simulink model "hybridperes (2)"  (R2019a)
settings: Solver=VariableStepAuto  StartTime=0.0  StopTime=10.0  RelTol=1e-3
libraries: powerlib x28, re_lib x2, powerlib_meascontrol x2
settings Model: Creator=USER  LastModifiedBy=USER

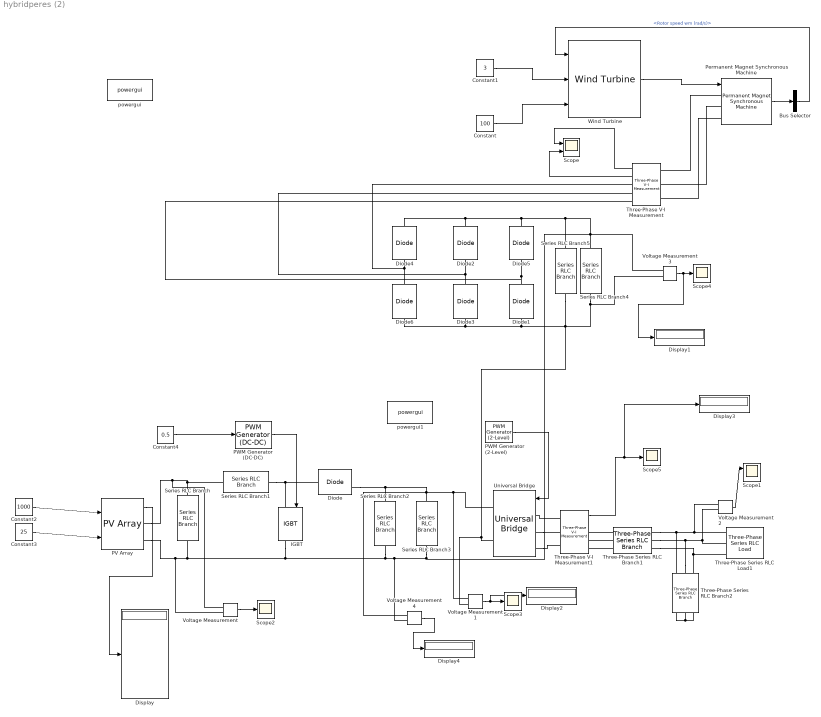
== system hybridperes (2) ==
  Bus Selector : BusSelector  OutputSignals=Rotor speed wm (rad/s)
  Constant : Constant  Value=100
  Constant1 : Constant  Value=3
  Constant2 : Constant  Value=1000
  Constant3 : Constant  Value=25
  Constant4 : Constant  Value=0.5
  Diode : powerlib/Power Electronics/Diode  Ron=0.001  Lon=0  Vf=0.8  IC=0  UseSnubber=0  Rs=500  Cs=250e-9  Measurements=on
      settings: SourceProductName=Simscape Electrical
  Diode{1..6} (6 alike) : powerlib/Power Electronics/Diode  Ron=0.001  Lon=0  Vf=0.8  IC=0  UseSnubber=0  Rs=500  Cs=250e-9  Measurements=off
      settings: SourceProductName=Simscape Electrical
  Display{,1..4} (5 alike) : Display
  IGBT : powerlib/Power Electronics/IGBT  Ron=0.001  Lon=0  Vf=1  Tf=1e-6  Tt=2e-6  IC=0  Rs=1e5  Cs=inf  Measurements=on
      settings: SourceProductName=Simscape Electrical
  PV Array : re_lib/Solar/PV Array  Npar=4  Nser=1  PlotType=array @ 1000 W/m2 & specified temperatures  S_vec="[ 1000  500  100 ]"  Temp_C_vec="[ 45 25  ]"  ModuleName=User-defined  PlotWhenSelected=off  Pm=213.15  Ncell=60  Voc=36.3  Isc=7.84  Vm=29  Im=7.35  beta_Voc_pc=-0.36099  alpha_Isc_pc=0.102  beta_Voc=-0.13104  alpha_Isc=0.0079968  IL=7.8654  I0=2.9273e-10  nI=0.98119  Rsh=313.0553  Rs=0.39381  BAL=on  Tc=1e-6  Tfilter=5e-5
      settings: SourceProductName=Simscape Electrical
  PWM Generator (2-Level) : powerlib_meascontrol/Pulse & Signal Generators/PWM Generator (2-Level)  ModulatorType=Three-phase bridge (6 pulses)  ModulatorMode=Unsynchronized  Fc=27*50*3  Pc=90  nF=27  MinMax="[ -1  1 ]"  SamplingTechnique=Natural  ModulatingSignals=on  m=0.8  Freq=50  Phase=0  Ts=0  ShowCarrierOutport=off
  PWM Generator (DC-DC) : powerlib_meascontrol/Pulse & Signal Generators/PWM Generator (DC-DC)  Fsw=5000  Ts=0
      settings: SourceProductName=Simscape Electrical
  Permanent Magnet Synchronous Machine : powerlib/Machines/Permanent Magnet Synchronous Machine  NbPhases=3  FluxDistribution=Sinusoidal  RotorType=Round  MechanicalLoad=Torque Tm  PresetModel=No  ShowDetailedParameters=on  MeasurementBus=off  Resistance=0.0485  Inductance=8.5e-3  dqInductances=[8.5e-3,8.5e-3]  La=0.000395  MachineConstant=Flux linkage established by magnets (V.s)  Flux=0.1194  VoltageCst=86.6271  TorqueCst=0.7164  Flat=120  Mechanical=[0.0027 0.0004924 4 0]  PolePairs=4  InitialConditions=[0,0, 0,0]  InitialConditions5ph=[0 0 0 0 0 0]  TsPowergui=0  TsBlock=-1  RefAngle=90 degrees behind phase A axis (modified Park)
  Scope : Scope  NumInputPorts=2
  Scope1 : Scope  NumInputPorts=2
  Scope{2..5} (4 alike) : Scope
  Series RLC Branch : powerlib/Elements/Series RLC Branch  LConnTagsString=__new0  RConnTagsString=__new0  BranchType=C  Resistance=1  Inductance=1e-3  SetiL0=off  InitialCurrent=0  Capacitance=0.5  Setx0=off  InitialVoltage=0  Measurements=None
      settings: SourceProductName=Simscape Electrical
  Series RLC Branch1 : powerlib/Elements/Series RLC Branch  LConnTagsString=__new0  RConnTagsString=__new0  BranchType=L  Resistance=1  Inductance=160e-6  SetiL0=off  InitialCurrent=0  Capacitance=1e-6  Setx0=off  InitialVoltage=0  Measurements=None
      settings: SourceProductName=Simscape Electrical
  Series RLC Branch2 : powerlib/Elements/Series RLC Branch  LConnTagsString=__new0  RConnTagsString=__new0  BranchType=C  Resistance=1  Inductance=1e-3  SetiL0=off  InitialCurrent=0  Capacitance=83e-3  Setx0=off  InitialVoltage=0  Measurements=None
      settings: SourceProductName=Simscape Electrical
  Series RLC Branch3 : powerlib/Elements/Series RLC Branch  LConnTagsString=__new0  RConnTagsString=__new0  BranchType=R  Resistance=2  Inductance=1e-3  SetiL0=off  InitialCurrent=0  Capacitance=1e-6  Setx0=off  InitialVoltage=0  Measurements=None
      settings: SourceProductName=Simscape Electrical
  Series RLC Branch4 : powerlib/Elements/Series RLC Branch  LConnTagsString=__new0  RConnTagsString=__new0  BranchType=R  Resistance=1  Inductance=1e-3  SetiL0=off  InitialCurrent=0  Capacitance=1e-6  Setx0=off  InitialVoltage=0  Measurements=None
      settings: SourceProductName=Simscape Electrical
  Series RLC Branch5 : powerlib/Elements/Series RLC Branch  LConnTagsString=__new0  RConnTagsString=__new0  BranchType=C  Resistance=1  Inductance=1e-3  SetiL0=off  InitialCurrent=0  Capacitance=10e-3  Setx0=off  InitialVoltage=0  Measurements=None
      settings: SourceProductName=Simscape Electrical
  Three-Phase Series RLC Branch1 : powerlib/Elements/Three-Phase Series RLC Branch  LConnTagsString=A|B|C  RConnTagsString=A|B|C  BranchType=L  Resistance=1  Inductance=0.001023  Capacitance=1e-6  Measurements=None
      settings: SourceProductName=Simscape Electrical
  Three-Phase Series RLC Branch2 : powerlib/Elements/Three-Phase Series RLC Branch  LConnTagsString=A|B|C  RConnTagsString=A|B|C  BranchType=C  Resistance=1  Inductance=1e-3  Capacitance=0.008456  Measurements=None
      settings: SourceProductName=Simscape Electrical
  Three-Phase Series RLC Load1 : powerlib/Elements/Three-Phase Series RLC Load  LConnTagsString=A|B|C  Configuration=Y (grounded)  NominalVoltage=1000  Vabc=[1e3 1e3 1e3]  Vabcp=[1e3 1e3 1e3]  NominalFrequency=50  UnbalancedPower=off  ActivePower=10e3  InductivePower=0  CapacitivePower=0  Pabc=[10e3 9e3 11e3]  QLabc=[100 90 110]  QCabc=[100 90 110]  Pabcp=[10e3 9e3 11e3]  QLabcp=[100 90 110]  QCabcp=[100 90 110]  Measurements=None  LoadType=constant Z
      settings: SourceProductName=Simscape Electrical
  Three-Phase V-I Measurement : powerlib/Measurements/Three-Phase V-I Measurement  VoltageMeasurement=phase-to-phase  SetLabelV=off  LabelV=Vabc  Vpu=off  VpuLL=off  CurrentMeasurement=yes  SetLabelI=off  LabelI=Iabc  Ipu=off  Pbase=100e6  Vbase=500e3  OutputType=Complex  PhasorSimulation=off  PSBequivalent=0
      settings: SourceProductName=Simscape Electrical
  Three-Phase V-I Measurement1 : powerlib/Measurements/Three-Phase V-I Measurement  VoltageMeasurement=phase-to-ground  SetLabelV=off  LabelV=Vabc  Vpu=off  VpuLL=off  CurrentMeasurement=yes  SetLabelI=off  LabelI=Iabc  Ipu=off  Pbase=100e6  Vbase=500e3  OutputType=Complex  PhasorSimulation=off  PSBequivalent=0
      settings: SourceProductName=Simscape Electrical
  Universal Bridge : powerlib/Power Electronics/Universal Bridge  Arms=3  SnubberResistance=1e5  SnubberCapacitance=inf  Device=IGBT / Diodes  Ron=1e-3  Lon=0  ForwardVoltages="[  0  0  ]"  ForwardVoltage=0  GTOparameters=[ 10e-6 , 20e-6 ]  IGBTparameters=[ 1e-6 , 2e-6 ]  Measurements=None  Measurements_2=None  converterType=Rectifier
      settings: SourceProductName=Simscape Electrical
  Voltage Measurement{,1..4} (5 alike) : powerlib/Measurements/Voltage Measurement  PhasorSimulation=off  OutputType=Complex  PSBequivalent=0
      settings: SourceProductName=Simscape Electrical
  Wind Turbine : re_lib/Wind Generation/Wind Turbine  Pnom=1.5e6  Pelec_base=1.5e6/0.9  wind_base=12  P_wind_base=0.73  speed_nom=1.2  pitch_angle=0  c1_c6="[0.51763          116          0.4            5           21     0.006795]"  cp_nom=0.48  lambda_nom=8.1
      settings: SourceProductName=Simscape Electrical  SourceProductBaseCode=PS
  powergui : powerlib/powergui  Priority=1  SimulationMode=Discrete  SampleTime=50e-6  frequency=60  Iterations=50  frequencyindice=0  Pbase=100e6  ErrMax=1e-4  UnitsV=kV  UnitsW=MW  buscounter=0  FunctionMessages=off  echomessages=off  EnableUseOfTLC=off  CurrentSourceSwitches=off  DisableSnubberDevices=off  DisableRonSwitches=off  DisableVfSwitches=off  DisplayEquations=off  AutomaticDiscreteSolvers=off  SolverType=Tustin/Backward Euler (TBE)  Interpol=off  ExternalGateDelay=off  methode=off  Ts=100  x0status=blocks  SPID=on  SwTol=0  HookPort=off  NonlinearTolerance=0  nMaxIteration=15  ContinueOnMaxIteration=off  RestoreLinks=warning  ResistiveCurrentMeasurement=off  Frange=[0:2:500]  Ylog=off  Xlog=on  ShowGrid=off  save=off  variable=ZData  structure=0  ZoomFFT=off  StartTime=0.0  cycles=1  DisplayStyle=1  fundamental=60  FreqAxis=off  MaxFrequency=1000  frequencyindicesteady=1  RmsSteady=1  display=off
      settings: SourceProductName=Simscape Electrical
  powergui1 : powerlib/powergui  Priority=1  SimulationMode=Discrete  SampleTime=5e-6  frequency=60  Iterations=50  frequencyindice=0  Pbase=100e6  ErrMax=1e-4  UnitsV=kV  UnitsW=MW  buscounter=0  FunctionMessages=off  echomessages=off  EnableUseOfTLC=off  CurrentSourceSwitches=off  DisableSnubberDevices=off  DisableRonSwitches=off  DisableVfSwitches=off  DisplayEquations=off  AutomaticDiscreteSolvers=off  SolverType=Tustin/Backward Euler (TBE)  Interpol=off  ExternalGateDelay=off  methode=off  Ts=100  x0status=blocks  SPID=on  SwTol=0  HookPort=off  NonlinearTolerance=0  nMaxIteration=15  ContinueOnMaxIteration=off  RestoreLinks=warning  ResistiveCurrentMeasurement=off  Frange=[0:2:500]  Ylog=off  Xlog=on  ShowGrid=off  save=off  variable=ZData  structure=0  ZoomFFT=off  StartTime=0.0  cycles=1  DisplayStyle=1  fundamental=60  FreqAxis=off  MaxFrequency=1000  frequencyindicesteady=1  RmsSteady=1  display=off
      settings: SourceProductName=Simscape Electrical
  wires:
  Constant/1 -> Wind Turbine/3
  Constant1/1 -> Wind Turbine/2
  Wind Turbine/1 -> Permanent Magnet Synchronous Machine/1
  Permanent Magnet Synchronous Machine/1 -> Bus Selector/1
  Bus Selector/1 -> Wind Turbine/1  "<Rotor speed wm (rad/s)>"
  Three-Phase V-I Measurement/1 -> Scope/1
  Three-Phase V-I Measurement/2 -> Scope/2
  Voltage Measurement/1 -> Scope2/1
  PWM Generator (2-Level)/1 -> Universal Bridge/1
  Voltage Measurement2/1 -> Scope1/1
  PV Array/1 -> Display/1
  Constant4/1 -> PWM Generator (DC-DC)/1
  Voltage Measurement1/1 -> Display2/1, Scope3/1
  PWM Generator (DC-DC)/1 -> IGBT/1
  Constant2/1 -> PV Array/1
  Constant3/1 -> PV Array/2
  Voltage Measurement3/1 -> Display1/1, Scope4/1
  Three-Phase V-I Measurement1/1 -> Display3/1, Scope5/1
  Voltage Measurement4/1 -> Display4/1
  connections:
  Diode/LConn1 -- Series RLC Branch1/RConn1 -- IGBT/LConn1
  Three-Phase Series RLC Load1/LConn1 -- Three-Phase Series RLC Branch1/RConn1 -- Three-Phase Series RLC Branch2/LConn1 -- Voltage Measurement2/LConn1
  Three-Phase Series RLC Branch2/LConn2 -- Three-Phase Series RLC Branch1/RConn2 -- Voltage Measurement2/LConn2 -- Three-Phase Series RLC Load1/LConn2
  Three-Phase Series RLC Branch2/RConn2 -- Three-Phase Series RLC Branch2/RConn1 -- Three-Phase Series RLC Branch2/RConn3
  Three-Phase Series RLC Load1/LConn3 -- Three-Phase Series RLC Branch1/RConn3 -- Three-Phase Series RLC Branch2/LConn3
  Diode4/RConn1 -- Voltage Measurement4/LConn2 -- Series RLC Branch2/RConn1 -- PV Array/RConn2 -- Voltage Measurement/LConn2 -- Series RLC Branch/RConn1 -- IGBT/RConn1 -- Series RLC Branch3/RConn1 -- Voltage Measurement3/LConn1 -- Series RLC Branch4/LConn1 -- Series RLC Branch5/LConn1 -- Diode5/RConn1 -- Diode2/RConn1
  Series RLC Branch/LConn1 -- PV Array/RConn1 -- Voltage Measurement/LConn1 -- Series RLC Branch1/LConn1
  Three-Phase Series RLC Branch1/LConn2 -- Three-Phase V-I Measurement1/RConn2
  Universal Bridge/LConn3 -- Three-Phase V-I Measurement1/LConn3
  Three-Phase Series RLC Branch1/LConn3 -- Three-Phase V-I Measurement1/RConn3
  Three-Phase V-I Measurement1/LConn1 -- Universal Bridge/LConn1
  Three-Phase Series RLC Branch1/LConn1 -- Three-Phase V-I Measurement1/RConn1
  Universal Bridge/LConn2 -- Three-Phase V-I Measurement1/LConn2
  Permanent Magnet Synchronous Machine/LConn1 -- Three-Phase V-I Measurement/LConn1
  Permanent Magnet Synchronous Machine/LConn2 -- Three-Phase V-I Measurement/LConn2
  Permanent Magnet Synchronous Machine/LConn3 -- Three-Phase V-I Measurement/LConn3
  Diode1/RConn1 -- Diode5/LConn1 -- Three-Phase V-I Measurement/RConn3
  Diode3/RConn1 -- Three-Phase V-I Measurement/RConn2 -- Diode2/LConn1
  Diode6/RConn1 -- Three-Phase V-I Measurement/RConn1 -- Diode4/LConn1
  Diode6/LConn1 -- Series RLC Branch5/RConn1 -- Universal Bridge/RConn2 -- Voltage Measurement1/LConn2 -- Series RLC Branch4/RConn1 -- Voltage Measurement3/LConn2 -- Diode1/LConn1 -- Diode3/LConn1
  Series RLC Branch2/LConn1 -- Diode/RConn1 -- Voltage Measurement1/LConn1 -- Universal Bridge/RConn1 -- Voltage Measurement4/LConn1 -- Series RLC Branch3/LConn1
